simulink model "Controller"  (R2018a)
settings: Solver=VariableStepAuto  StartTime=0.0  StopTime=10.0  RelTol=1e-3
values from neighbouring files (symbols this model uses):
  q1_0 = 45*pi/180    (= 0.785398163397)    [Ableiten.m]    (also in Parameter.m = initConds.alpha1_0)
  q1_dot_0 = 0    [Ableiten.m]    (also in Parameter.m)
  q2_0 = 45*pi/180    (= 0.785398163397)    [Ableiten.m]    (also in Parameter.m = initConds.alpha2_0)
  q2_dot_0 = 0    [Ableiten.m]    (also in Parameter.m)
settings Model: Creator=MJ  LastModifiedBy=MJ

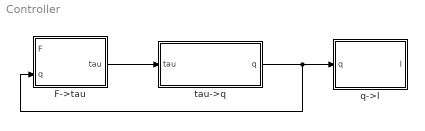
== system Controller ==
  F->tau : MATLAB Function  TreatAsAtomicUnit=on
  q->l : MATLAB Function  TreatAsAtomicUnit=on
  tau->q : Subsystem
  wires:
  F->tau/1(tau) -> tau->q/1(tau)
  tau->q/1(q) -> F->tau/2(q), q->l/1(q)

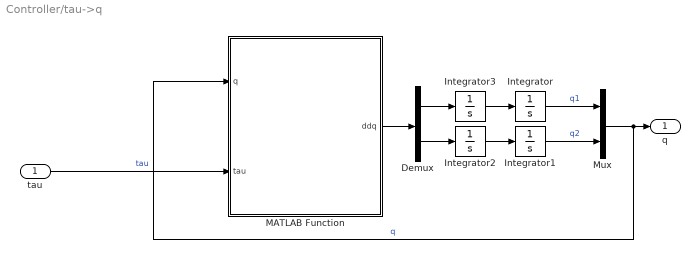
== system Controller/tau->q ==
  tau : Inport
  Demux : Demux  Outputs=2
  Integrator : Integrator  InitialCondition=q1_0
  Integrator1 : Integrator  InitialCondition=q2_0
  Integrator2 : Integrator  InitialCondition=q2_dot_0
  Integrator3 : Integrator  InitialCondition=q1_dot_0
  MATLAB Function : MATLAB Function  TreatAsAtomicUnit=on
  Mux : Mux  Inputs=2
  q : Outport
  wires:
  Integrator3/1 -> Integrator/1
  tau/1 -> MATLAB Function/2(tau)  "tau"
  Integrator2/1 -> Integrator1/1
  Integrator/1 -> Mux/1  "q1"
  Integrator1/1 -> Mux/2  "q2"
  Mux/1 -> MATLAB Function/1(q), q/1  "q"
  MATLAB Function/1(ddq) -> Demux/1
  Demux/1 -> Integrator3/1
  Demux/2 -> Integrator2/1

== matlab function Controller/q->l ==
  data: q input; l output
function l = fcn(q)

q1 = q(1);
q2 = q(2);

l = [sqrt((sin(q1).*(1.0./1.0e1)-3.707106781186548e-1).^2+(cos(q1).*(1.0./1.0e1)-sqrt(2.0).*(1.0./2.0e1)).^2);sqrt((sin(q2).*(1.0./1.0e1)-3.707106781186548e-1).^2+(cos(q2).*(1.0./1.0e1)-sqrt(2.0).*(1.0./2.0e1)).^2)];

== matlab function Controller/F->tau ==
  data: F input; tau output; q input
function tau = fcn(F,q)

q1 = q(1);
q2 = q(2);

J = [
    [ -(L0*(2*Lp*cos(q1) + 2^(1/2)*L0*cos(q1) - 2^(1/2)*L0*sin(q1)))/((2*Lp + 2^(1/2)*L0 - 2*L0*sin(q1))^2 + L0^2*(2*cos(q1) - 2^(1/2))^2)^(1/2),                                                                                                                                          0];
    [                                                                                                                                          0, -(L0*(2*Lp*cos(q2) + 2^(1/2)*L0*cos(q2) - 2^(1/2)*L0*sin(q2)))/((2*Lp + 2^(1/2)*L0 - 2*L0*sin(q2))^2 + L0^2*(2*cos(q2) - 2^(1/2))^2)^(1/2)]
    ];

tau = -J'*F;

== matlab function Controller/tau->q/MATLAB Function ==
  data: q input; ddq output; tau input
function ddq = fcn(q,tau)

ddq1 = (2^(1/2)*L0^2*k1*sin(q1 + q2)*(2*d10 - 2^(1/2)*(-L0^2*(cos(q1 + q2) - 1))^(1/2)))/(8*(-L0^2*(cos(q1 + q2) - 1))^(1/2)) - (2^(1/2)*L0^2*k2*(d20 - 2^(1/2)*(L0^2*(2*sin(pi/9) + cos(q1 + q2 + (2*pi)/9) - 2*sin(q1 + q2 + pi/9) - cos(q1 + q2) + 2))^(1/2))*(2*cos(q1 + q2 + pi/9) + sin(q1 + q2 + (2*pi)/9) - sin(q1 + q2)))/(2*(L0^2*(2*sin(pi/9) + cos(q1 + q2 + (2*pi)/9) - 2*sin(q1 + q2 + pi/9) - cos(q1 + q2) + 2))^(1/2))/I;
ddq2 = (2^(1/2)*L0^2*k1*sin(q1 + q2)*(2*d10 - 2^(1/2)*(-L0^2*(cos(q1 + q2) - 1))^(1/2)))/(8*(-L0^2*(cos(q1 + q2) - 1))^(1/2)) - (2^(1/2)*L0^2*k2*(d20 - 2^(1/2)*(L0^2*(2*sin(pi/9) + cos(q1 + q2 + (2*pi)/9) - 2*sin(q1 + q2 + pi/9) - cos(q1 + q2) + 2))^(1/2))*(2*cos(q1 + q2 + pi/9) + sin(q1 + q2 + (2*pi)/9) - sin(q1 + q2)))/(2*(L0^2*(2*sin(pi/9) + cos(q1 + q2 + (2*pi)/9) - 2*sin(q1 + q2 + pi/9) - cos(q1 + q2) + 2))^(1/2))/I;

ddq = [ddq1;ddq2];
